simulink model "Last_Model_Interior_team"  (R2017b)
settings: Solver=VariableStepAuto  SolverName=FixedStepDiscrete  StartTime=0.0  StopTime=10  FixedStep=1e-6
PreLoadFcn:
  | %% Motor Parameters
  | Rs=6.9*10^-3;
  | Ld=220*10^-6;
  | Lq=265.4*10^-6;
  | Pm=87.78*10^-3;
  | P=4;
  | b=0.0019;
  | J=0.13;
  | f=50;
  | P_Rated=100000;
  | N_Rated=6320;
  | N_max=30000;
  | Tfl=P_Rated/(N_Rated*(2*pi/60));
  | Tl=0;
  | 
  | %% hardware impl
  | Vdc=340;
  | clocking=100;
  | fs=10000;
  | Ts=1/fs;
  | Irated=500;
  | Imax=500;
  | Id_MAX=-(Pm/Ld);
  | I_Limit=Irated;
  | I_fw=I_Limit;
  | Vmax=Vdc/sqrt(3);
  | update=2;
  | 
  | 
  | %% Inverter
  | Vdc=340;
  | deadtime=1e-6;
  | 
  | 
  | 
  | %% Tuning OF Id_Pole_Placment
  | zeta_Id=0.707;
  | Gamma_Id=0.9;
  | Wn_Id=(1/(1-Gamma_Id))*(Rs/Ld);
  | Kc_Id=(2*zeta_Id*Ld*Wn_Id)-Rs;
  | TAW_Id=((2*zeta_Id*Wn_Id*Ld)-Rs)/(Ld*Wn_Id*Wn_Id);
  | 
  | %% Tuning OF Iq_Pole_Placment
  | zeta_Iq=0.707;
  | Gamma_Iq=0.9;
  | Wn_Iq=(1/(1-Gamma_Iq))*(Rs/Lq);
  | Kc_Iq=(2*zeta_Iq*Lq*Wn_Iq)-Rs;
  | TAW_Iq=((2*zeta_Iq*Wn_Iq*Lq)-Rs)/(Lq*Wn_Iq*Wn_Iq);
  | 
  | 
  | 
  | %% Tuning of PI Using Symmetric Optimum For q phase
  | Tc=(1/fs)/update;
  | A=8;
  | Kp_SO_q=Lq/(A*(Tc)*1.5);
  | Ki_SO_q=1/((A^2)*1.5*Tc);
  | %% Tuning of PI Using Symmetric Optimum For d phase
  | Kp_SO_d=Ld/(A*(Tc)*1.5);
  | Ki_SO_d=1/((A^2)*1.5*Tc);
  | 
  | ... (+20 lines)
InitFcn:
  | %% Motor Parameters
  | Rs=6.9*10^-3;
  | Ld=220*10^-6;
  | Lq=265.4*10^-6;
  | Pm=87.78*10^-3;
  | P=4;
  | b=0.0019;
  | J=0.13;
  | f=50;
  | P_Rated=100000;
  | N_Rated=6320;
  | N_max=30000;
  | Tfl=P_Rated/(N_Rated*(2*pi/60));
  | Tl=0;
  | 
  | %% hardware impl
  | Vdc=340;
  | clocking=100;
  | fs=10000;
  | Ts=1/fs;
  | Irated=500;
  | Imax=500;
  | Id_MAX=-(Pm/Ld);
  | I_Limit=Irated;
  | I_fw=I_Limit;
  | Vmax=Vdc/sqrt(3);
  | update=2;
  | 
  | %% Inverter
  | Vdc=340;
  | deadtime=1e-6;
  | 
  | 
  | 
  | %% Tuning OF Id_Pole_Placment
  | zeta_Id=0.707;
  | Gamma_Id=0.9;
  | Wn_Id=(1/(1-Gamma_Id))*(Rs/Ld);
  | Kc_Id=(2*zeta_Id*Ld*Wn_Id)-Rs;
  | TAW_Id=((2*zeta_Id*Wn_Id*Ld)-Rs)/(Ld*Wn_Id*Wn_Id);
  | 
  | %% Tuning OF Iq_Pole_Placment
  | zeta_Iq=0.707;
  | Gamma_Iq=0.9;
  | Wn_Iq=(1/(1-Gamma_Iq))*(Rs/Lq);
  | Kc_Iq=(2*zeta_Iq*Lq*Wn_Iq)-Rs;
  | TAW_Iq=((2*zeta_Iq*Wn_Iq*Lq)-Rs)/(Lq*Wn_Iq*Wn_Iq);
  | 
  | 
  | 
  | %% Tuning of PI Using Symmetric Optimum For q phase
  | Tc=(1/fs)/update;
  | A=8;
  | Kp_SO_q=Lq/(A*(Tc)*1.5);
  | Ki_SO_q=1/((A^2)*1.5*Tc);
  | %% Tuning of PI Using Symmetric Optimum For d phase
  | Kp_SO_d=Ld/(A*(Tc)*1.5);
  | Ki_SO_d=1/((A^2)*1.5*Tc);
  | 
  | 
  | ... (+19 lines)
undefined symbols (not defined in the file): DiscIntNeverNeededParam, magnitude
libraries: simulink x81, powerlib x14
(part 3 of 4)

== system Last_Model_Interior_team/Switching/30_deg_Dpwm/Sector2 ==
  Vabc : Inport
  Enable : EnablePort
  Compare To Zero : simulink/Logic and Bit Operations/Compare To Zero  relop=<  OutDataTypeStr=boolean
  Compare To Zero1 : simulink/Logic and Bit Operations/Compare To Zero  relop=>=  OutDataTypeStr=boolean
  Demux : Demux  Outputs=3
  Enabled Subsystem : Subsystem  TreatAsAtomicUnit=on
  Enabled Subsystem1 : Subsystem  TreatAsAtomicUnit=on
  Merge : Merge
  Terminator : Terminator
  Terminator1 : Terminator
  Out1 : Outport
  wires:
  Demux/1 -> Terminator/1
  Compare To Zero/1 -> Enabled Subsystem/Enable
  Compare To Zero1/1 -> Enabled Subsystem1/Enable
  Enabled Subsystem/1(Out1) -> Merge/1
  Enabled Subsystem1/1(Out1) -> Merge/2
  Merge/1 -> Out1/1
  Vabc/1 -> Enabled Subsystem1/1(Vabc), Enabled Subsystem/1(Vabc), Demux/1
  Demux/2 -> Compare To Zero1/1, Compare To Zero/1
  Demux/3 -> Terminator1/1

== system Last_Model_Interior_team/Switching/30_deg_Dpwm/Sector3 ==
  Vabc : Inport
  Enable : EnablePort
  Compare To Zero : simulink/Logic and Bit Operations/Compare To Zero  relop=<  OutDataTypeStr=boolean
  Compare To Zero1 : simulink/Logic and Bit Operations/Compare To Zero  relop=>=  OutDataTypeStr=boolean
  Demux : Demux  Outputs=3
  Enabled Subsystem : Subsystem  TreatAsAtomicUnit=on
  Enabled Subsystem1 : Subsystem  TreatAsAtomicUnit=on
  Merge : Merge
  Terminator : Terminator
  Terminator1 : Terminator
  Out1 : Outport
  wires:
  Demux/2 -> Terminator1/1
  Demux/3 -> Compare To Zero/1, Compare To Zero1/1
  Vabc/1 -> Demux/1, Enabled Subsystem/1(Vabc), Enabled Subsystem1/1(Vabc)
  Merge/1 -> Out1/1
  Enabled Subsystem1/1(Out1) -> Merge/2
  Enabled Subsystem/1(Out1) -> Merge/1
  Compare To Zero1/1 -> Enabled Subsystem1/Enable
  Compare To Zero/1 -> Enabled Subsystem/Enable
  Demux/1 -> Terminator/1

== system Last_Model_Interior_team/Switching/30_deg_Dpwm/Sector4 ==
  Vabc : Inport
  Enable : EnablePort
  Compare To Zero : simulink/Logic and Bit Operations/Compare To Zero  relop=<  OutDataTypeStr=boolean
  Compare To Zero1 : simulink/Logic and Bit Operations/Compare To Zero  relop=>=  OutDataTypeStr=boolean
  Demux : Demux  Outputs=3
  Enabled Subsystem : Subsystem  TreatAsAtomicUnit=on
  Enabled Subsystem1 : Subsystem  TreatAsAtomicUnit=on
  Merge : Merge
  Terminator : Terminator
  Terminator1 : Terminator
  Out1 : Outport
  wires:
  Demux/3 -> Terminator/1
  Demux/1 -> Compare To Zero/1, Compare To Zero1/1
  Compare To Zero/1 -> Enabled Subsystem/Enable
  Compare To Zero1/1 -> Enabled Subsystem1/Enable
  Enabled Subsystem/1(Out1) -> Merge/1
  Enabled Subsystem1/1(Out1) -> Merge/2
  Merge/1 -> Out1/1
  Vabc/1 -> Enabled Subsystem/1(Vabc), Enabled Subsystem1/1(Vabc), Demux/1
  Demux/2 -> Terminator1/1

== system Last_Model_Interior_team/Switching/30_deg_Dpwm/Sector5 ==
  Vabc : Inport
  Enable : EnablePort
  Compare To Zero : simulink/Logic and Bit Operations/Compare To Zero  relop=<  OutDataTypeStr=boolean
  Compare To Zero1 : simulink/Logic and Bit Operations/Compare To Zero  relop=>=  OutDataTypeStr=boolean
  Demux : Demux  Outputs=3
  Enabled Subsystem : Subsystem  TreatAsAtomicUnit=on
  Enabled Subsystem1 : Subsystem  TreatAsAtomicUnit=on
  Merge : Merge
  Terminator : Terminator
  Terminator1 : Terminator
  Out1 : Outport
  wires:
  Demux/1 -> Terminator1/1
  Demux/2 -> Compare To Zero1/1, Compare To Zero/1
  Vabc/1 -> Demux/1, Enabled Subsystem1/1(Vabc), Enabled Subsystem/1(Vabc)
  Merge/1 -> Out1/1
  Enabled Subsystem1/1(Out1) -> Merge/2
  Enabled Subsystem/1(Out1) -> Merge/1
  Compare To Zero1/1 -> Enabled Subsystem1/Enable
  Compare To Zero/1 -> Enabled Subsystem/Enable
  Demux/3 -> Terminator/1

== system Last_Model_Interior_team/Switching/30_deg_Dpwm/Sector6 ==
  Vabc : Inport
  Enable : EnablePort
  Compare To Zero : simulink/Logic and Bit Operations/Compare To Zero  relop=<  OutDataTypeStr=boolean
  Compare To Zero1 : simulink/Logic and Bit Operations/Compare To Zero  relop=>=  OutDataTypeStr=boolean
  Demux : Demux  Outputs=3
  Enabled Subsystem : Subsystem  TreatAsAtomicUnit=on
  Enabled Subsystem1 : Subsystem  TreatAsAtomicUnit=on
  Merge : Merge
  Terminator : Terminator
  Terminator1 : Terminator
  Out1 : Outport
  wires:
  Demux/3 -> Compare To Zero/1, Compare To Zero1/1
  Compare To Zero/1 -> Enabled Subsystem/Enable
  Compare To Zero1/1 -> Enabled Subsystem1/Enable
  Enabled Subsystem/1(Out1) -> Merge/1
  Enabled Subsystem1/1(Out1) -> Merge/2
  Merge/1 -> Out1/1
  Vabc/1 -> Enabled Subsystem/1(Vabc), Enabled Subsystem1/1(Vabc), Demux/1
  Demux/1 -> Terminator1/1
  Demux/2 -> Terminator/1

== system Last_Model_Interior_team/Switching/60deg_+30_shifted/Sector1 ==
  Vabc : Inport
  Enable : EnablePort
  Compare To Zero : simulink/Logic and Bit Operations/Compare To Zero  relop=<  OutDataTypeStr=boolean
  Compare To Zero1 : simulink/Logic and Bit Operations/Compare To Zero  relop=>=  OutDataTypeStr=boolean
  Demux : Demux  Outputs=3
  Enabled Subsystem : Subsystem  TreatAsAtomicUnit=on
  Enabled Subsystem1 : Subsystem  TreatAsAtomicUnit=on
  Merge : Merge
  Terminator : Terminator
  Terminator1 : Terminator
  Out1 : Outport
  wires:
  Compare To Zero/1 -> Enabled Subsystem/Enable
  Compare To Zero1/1 -> Enabled Subsystem1/Enable
  Enabled Subsystem/1(Out1) -> Merge/1
  Enabled Subsystem1/1(Out1) -> Merge/2
  Merge/1 -> Out1/1
  Vabc/1 -> Enabled Subsystem/1(Vabc), Enabled Subsystem1/1(Vabc), Demux/1
  Demux/1 -> Compare To Zero1/1, Compare To Zero/1
  Demux/2 -> Terminator/1
  Demux/3 -> Terminator1/1

== system Last_Model_Interior_team/Switching/60deg_+30_shifted/Sector2 ==
  Vabc : Inport
  Enable : EnablePort
  Compare To Zero : simulink/Logic and Bit Operations/Compare To Zero  relop=<  OutDataTypeStr=boolean
  Compare To Zero1 : simulink/Logic and Bit Operations/Compare To Zero  relop=>=  OutDataTypeStr=boolean
  Demux : Demux  Outputs=3
  Enabled Subsystem : Subsystem  TreatAsAtomicUnit=on
  Enabled Subsystem1 : Subsystem  TreatAsAtomicUnit=on
  Merge : Merge
  Terminator : Terminator
  Terminator1 : Terminator
  Out1 : Outport
  wires:
  Demux/3 -> Terminator1/1
  Demux/2 -> Compare To Zero1/1, Compare To Zero/1
  Vabc/1 -> Demux/1, Enabled Subsystem/1(Vabc), Enabled Subsystem1/1(Vabc)
  Merge/1 -> Out1/1
  Enabled Subsystem1/1(Out1) -> Merge/2
  Enabled Subsystem/1(Out1) -> Merge/1
  Compare To Zero1/1 -> Enabled Subsystem1/Enable
  Compare To Zero/1 -> Enabled Subsystem/Enable
  Demux/1 -> Terminator/1

== system Last_Model_Interior_team/Switching/60deg_+30_shifted/Sector3 ==
  Vabc : Inport
  Enable : EnablePort
  Compare To Zero : simulink/Logic and Bit Operations/Compare To Zero  relop=<  OutDataTypeStr=boolean
  Compare To Zero1 : simulink/Logic and Bit Operations/Compare To Zero  relop=>=  OutDataTypeStr=boolean
  Demux : Demux  Outputs=3
  Enabled Subsystem : Subsystem  TreatAsAtomicUnit=on
  Enabled Subsystem1 : Subsystem  TreatAsAtomicUnit=on
  Merge : Merge
  Terminator : Terminator
  Terminator1 : Terminator
  Out1 : Outport
  wires:
  Demux/1 -> Terminator/1
  Compare To Zero/1 -> Enabled Subsystem/Enable
  Compare To Zero1/1 -> Enabled Subsystem1/Enable
  Enabled Subsystem/1(Out1) -> Merge/1
  Enabled Subsystem1/1(Out1) -> Merge/2
  Merge/1 -> Out1/1
  Vabc/1 -> Enabled Subsystem1/1(Vabc), Enabled Subsystem/1(Vabc), Demux/1
  Demux/3 -> Compare To Zero1/1, Compare To Zero/1
  Demux/2 -> Terminator1/1

== system Last_Model_Interior_team/Switching/60deg_+30_shifted/Sector4 ==
  Vabc : Inport
  Enable : EnablePort
  Compare To Zero : simulink/Logic and Bit Operations/Compare To Zero  relop=<  OutDataTypeStr=boolean
  Compare To Zero1 : simulink/Logic and Bit Operations/Compare To Zero  relop=>=  OutDataTypeStr=boolean
  Demux : Demux  Outputs=3
  Enabled Subsystem : Subsystem  TreatAsAtomicUnit=on
  Enabled Subsystem1 : Subsystem  TreatAsAtomicUnit=on
  Merge : Merge
  Terminator : Terminator
  Terminator1 : Terminator
  Out1 : Outport
  wires:
  Demux/2 -> Terminator1/1
  Vabc/1 -> Demux/1, Enabled Subsystem1/1(Vabc), Enabled Subsystem/1(Vabc)
  Merge/1 -> Out1/1
  Enabled Subsystem1/1(Out1) -> Merge/2
  Enabled Subsystem/1(Out1) -> Merge/1
  Compare To Zero1/1 -> Enabled Subsystem1/Enable
  Compare To Zero/1 -> Enabled Subsystem/Enable
  Demux/1 -> Compare To Zero1/1, Compare To Zero/1
  Demux/3 -> Terminator/1

== system Last_Model_Interior_team/Switching/60deg_+30_shifted/Sector5 ==
  Vabc : Inport
  Enable : EnablePort
  Compare To Zero : simulink/Logic and Bit Operations/Compare To Zero  relop=<  OutDataTypeStr=boolean
  Compare To Zero1 : simulink/Logic and Bit Operations/Compare To Zero  relop=>=  OutDataTypeStr=boolean
  Demux : Demux  Outputs=3
  Enabled Subsystem : Subsystem  TreatAsAtomicUnit=on
  Enabled Subsystem1 : Subsystem  TreatAsAtomicUnit=on
  Merge : Merge
  Terminator : Terminator
  Terminator1 : Terminator
  Out1 : Outport
  wires:
  Demux/3 -> Terminator/1
  Compare To Zero/1 -> Enabled Subsystem/Enable
  Compare To Zero1/1 -> Enabled Subsystem1/Enable
  Enabled Subsystem/1(Out1) -> Merge/1
  Enabled Subsystem1/1(Out1) -> Merge/2
  Merge/1 -> Out1/1
  Vabc/1 -> Enabled Subsystem/1(Vabc), Enabled Subsystem1/1(Vabc), Demux/1
  Demux/2 -> Compare To Zero/1, Compare To Zero1/1
  Demux/1 -> Terminator1/1

== system Last_Model_Interior_team/Switching/60deg_+30_shifted/Sector6 ==
  Vabc : Inport
  Enable : EnablePort
  Compare To Zero : simulink/Logic and Bit Operations/Compare To Zero  relop=<  OutDataTypeStr=boolean
  Compare To Zero1 : simulink/Logic and Bit Operations/Compare To Zero  relop=>=  OutDataTypeStr=boolean
  Demux : Demux  Outputs=3
  Enabled Subsystem : Subsystem  TreatAsAtomicUnit=on
  Enabled Subsystem1 : Subsystem  TreatAsAtomicUnit=on
  Merge : Merge
  Terminator : Terminator
  Terminator1 : Terminator
  Out1 : Outport
  wires:
  Demux/1 -> Terminator1/1
  Vabc/1 -> Demux/1, Enabled Subsystem1/1(Vabc), Enabled Subsystem/1(Vabc)
  Merge/1 -> Out1/1
  Enabled Subsystem1/1(Out1) -> Merge/2
  Enabled Subsystem/1(Out1) -> Merge/1
  Compare To Zero1/1 -> Enabled Subsystem1/Enable
  Compare To Zero/1 -> Enabled Subsystem/Enable
  Demux/3 -> Compare To Zero1/1, Compare To Zero/1
  Demux/2 -> Terminator/1

== system Last_Model_Interior_team/Switching/60deg_-30_shifted/Sector1 ==
  Vabc : Inport
  Enable : EnablePort
  Compare To Zero : simulink/Logic and Bit Operations/Compare To Zero  relop=<  OutDataTypeStr=boolean
  Compare To Zero1 : simulink/Logic and Bit Operations/Compare To Zero  relop=>=  OutDataTypeStr=boolean
  Demux : Demux  Outputs=3
  Enabled Subsystem : Subsystem  TreatAsAtomicUnit=on
  Enabled Subsystem1 : Subsystem  TreatAsAtomicUnit=on
  Merge : Merge
  Terminator : Terminator
  Terminator1 : Terminator
  Out1 : Outport
  wires:
  Demux/3 -> Terminator1/1
  Demux/2 -> Terminator/1
  Demux/1 -> Compare To Zero/1, Compare To Zero1/1
  Vabc/1 -> Demux/1, Enabled Subsystem1/1(Vabc), Enabled Subsystem/1(Vabc)
  Merge/1 -> Out1/1
  Enabled Subsystem1/1(Out1) -> Merge/2
  Enabled Subsystem/1(Out1) -> Merge/1
  Compare To Zero1/1 -> Enabled Subsystem1/Enable
  Compare To Zero/1 -> Enabled Subsystem/Enable

== system Last_Model_Interior_team/Switching/60deg_-30_shifted/Sector2 ==
  Vabc : Inport
  Enable : EnablePort
  Compare To Zero : simulink/Logic and Bit Operations/Compare To Zero  relop=<  OutDataTypeStr=boolean
  Compare To Zero1 : simulink/Logic and Bit Operations/Compare To Zero  relop=>=  OutDataTypeStr=boolean
  Demux : Demux  Outputs=3
  Enabled Subsystem : Subsystem  TreatAsAtomicUnit=on
  Enabled Subsystem1 : Subsystem  TreatAsAtomicUnit=on
  Merge : Merge
  Terminator : Terminator
  Terminator1 : Terminator
  Out1 : Outport
  wires:
  Demux/1 -> Terminator/1
  Compare To Zero/1 -> Enabled Subsystem/Enable
  Compare To Zero1/1 -> Enabled Subsystem1/Enable
  Enabled Subsystem/1(Out1) -> Merge/1
  Enabled Subsystem1/1(Out1) -> Merge/2
  Merge/1 -> Out1/1
  Vabc/1 -> Enabled Subsystem1/1(Vabc), Enabled Subsystem/1(Vabc), Demux/1
  Demux/2 -> Compare To Zero/1, Compare To Zero1/1
  Demux/3 -> Terminator1/1

== system Last_Model_Interior_team/Switching/60deg_-30_shifted/Sector3 ==
  Vabc : Inport
  Enable : EnablePort
  Compare To Zero : simulink/Logic and Bit Operations/Compare To Zero  relop=<  OutDataTypeStr=boolean
  Compare To Zero1 : simulink/Logic and Bit Operations/Compare To Zero  relop=>=  OutDataTypeStr=boolean
  Demux : Demux  Outputs=3
  Enabled Subsystem : Subsystem  TreatAsAtomicUnit=on
  Enabled Subsystem1 : Subsystem  TreatAsAtomicUnit=on
  Merge : Merge
  Terminator : Terminator
  Terminator1 : Terminator
  Out1 : Outport
  wires:
  Demux/2 -> Terminator1/1
  Demux/3 -> Compare To Zero/1, Compare To Zero1/1
  Vabc/1 -> Demux/1, Enabled Subsystem/1(Vabc), Enabled Subsystem1/1(Vabc)
  Merge/1 -> Out1/1
  Enabled Subsystem1/1(Out1) -> Merge/2
  Enabled Subsystem/1(Out1) -> Merge/1
  Compare To Zero1/1 -> Enabled Subsystem1/Enable
  Compare To Zero/1 -> Enabled Subsystem/Enable
  Demux/1 -> Terminator/1

== system Last_Model_Interior_team/Switching/60deg_-30_shifted/Sector4 ==
  Vabc : Inport
  Enable : EnablePort
  Compare To Zero : simulink/Logic and Bit Operations/Compare To Zero  relop=<  OutDataTypeStr=boolean
  Compare To Zero1 : simulink/Logic and Bit Operations/Compare To Zero  relop=>=  OutDataTypeStr=boolean
  Demux : Demux  Outputs=3
  Enabled Subsystem : Subsystem  TreatAsAtomicUnit=on
  Enabled Subsystem1 : Subsystem  TreatAsAtomicUnit=on
  Merge : Merge
  Terminator : Terminator
  Terminator1 : Terminator
  Out1 : Outport
  wires:
  Demux/3 -> Terminator/1
  Demux/1 -> Compare To Zero/1, Compare To Zero1/1
  Compare To Zero/1 -> Enabled Subsystem/Enable
  Compare To Zero1/1 -> Enabled Subsystem1/Enable
  Enabled Subsystem/1(Out1) -> Merge/1
  Enabled Subsystem1/1(Out1) -> Merge/2
  Merge/1 -> Out1/1
  Vabc/1 -> Enabled Subsystem/1(Vabc), Enabled Subsystem1/1(Vabc), Demux/1
  Demux/2 -> Terminator1/1

== system Last_Model_Interior_team/Switching/60deg_-30_shifted/Sector5 ==
  Vabc : Inport
  Enable : EnablePort
  Compare To Zero : simulink/Logic and Bit Operations/Compare To Zero  relop=<  OutDataTypeStr=boolean
  Compare To Zero1 : simulink/Logic and Bit Operations/Compare To Zero  relop=>=  OutDataTypeStr=boolean
  Demux : Demux  Outputs=3
  Enabled Subsystem : Subsystem  TreatAsAtomicUnit=on
  Enabled Subsystem1 : Subsystem  TreatAsAtomicUnit=on
  Merge : Merge
  Terminator : Terminator
  Terminator1 : Terminator
  Out1 : Outport
  wires:
  Demux/1 -> Terminator1/1
  Demux/2 -> Compare To Zero1/1, Compare To Zero/1
  Vabc/1 -> Demux/1, Enabled Subsystem1/1(Vabc), Enabled Subsystem/1(Vabc)
  Merge/1 -> Out1/1
  Enabled Subsystem1/1(Out1) -> Merge/2
  Enabled Subsystem/1(Out1) -> Merge/1
  Compare To Zero1/1 -> Enabled Subsystem1/Enable
  Compare To Zero/1 -> Enabled Subsystem/Enable
  Demux/3 -> Terminator/1

== system Last_Model_Interior_team/Switching/60deg_-30_shifted/Sector6 ==
  Vabc : Inport
  Enable : EnablePort
  Compare To Zero : simulink/Logic and Bit Operations/Compare To Zero  relop=<  OutDataTypeStr=boolean
  Compare To Zero1 : simulink/Logic and Bit Operations/Compare To Zero  relop=>=  OutDataTypeStr=boolean
  Demux : Demux  Outputs=3
  Enabled Subsystem : Subsystem  TreatAsAtomicUnit=on
  Enabled Subsystem1 : Subsystem  TreatAsAtomicUnit=on
  Merge : Merge
  Terminator : Terminator
  Terminator1 : Terminator
  Out1 : Outport
  wires:
  Demux/2 -> Terminator/1
  Demux/3 -> Compare To Zero/1, Compare To Zero1/1
  Compare To Zero/1 -> Enabled Subsystem/Enable
  Compare To Zero1/1 -> Enabled Subsystem1/Enable
  Enabled Subsystem/1(Out1) -> Merge/1
  Enabled Subsystem1/1(Out1) -> Merge/2
  Merge/1 -> Out1/1
  Vabc/1 -> Enabled Subsystem/1(Vabc), Enabled Subsystem1/1(Vabc), Demux/1
  Demux/1 -> Terminator1/1

== system Last_Model_Interior_team/Switching/60deg_DPWM/Sector1 ==
  Vabc : Inport
  Enable : EnablePort
  Compare To Zero : simulink/Logic and Bit Operations/Compare To Zero  relop=<  OutDataTypeStr=boolean
  Compare To Zero1 : simulink/Logic and Bit Operations/Compare To Zero  relop=>=  OutDataTypeStr=boolean
  Demux : Demux  Outputs=3
  Enabled Subsystem : Subsystem  TreatAsAtomicUnit=on
  Enabled Subsystem1 : Subsystem  TreatAsAtomicUnit=on
  Merge : Merge
  Terminator : Terminator
  Terminator1 : Terminator
  Out1 : Outport
  wires:
  Enabled Subsystem/1(Out1) -> Merge/1
  Enabled Subsystem1/1(Out1) -> Merge/2
  Merge/1 -> Out1/1
  Vabc/1 -> Enabled Subsystem/1(Vabc), Enabled Subsystem1/1(Vabc), Demux/1
  Demux/1 -> Compare To Zero1/1, Compare To Zero/1
  Demux/2 -> Terminator/1
  Demux/3 -> Terminator1/1
  Compare To Zero1/1 -> Enabled Subsystem1/Enable
  Compare To Zero/1 -> Enabled Subsystem/Enable

== system Last_Model_Interior_team/Switching/60deg_DPWM/Sector2 ==
  Vabc : Inport
  Enable : EnablePort
  Compare To Zero : simulink/Logic and Bit Operations/Compare To Zero  relop=<  OutDataTypeStr=boolean
  Compare To Zero1 : simulink/Logic and Bit Operations/Compare To Zero  relop=>=  OutDataTypeStr=boolean
  Demux : Demux  Outputs=3
  Enabled Subsystem : Subsystem  TreatAsAtomicUnit=on
  Enabled Subsystem1 : Subsystem  TreatAsAtomicUnit=on
  Merge : Merge
  Terminator : Terminator
  Terminator1 : Terminator
  Out1 : Outport
  wires:
  Demux/3 -> Terminator1/1
  Demux/2 -> Compare To Zero1/1, Compare To Zero/1
  Vabc/1 -> Demux/1, Enabled Subsystem1/1(Vabc), Enabled Subsystem/1(Vabc)
  Merge/1 -> Out1/1
  Enabled Subsystem1/1(Out1) -> Merge/2
  Enabled Subsystem/1(Out1) -> Merge/1
  Compare To Zero1/1 -> Enabled Subsystem1/Enable
  Compare To Zero/1 -> Enabled Subsystem/Enable
  Demux/1 -> Terminator/1

== system Last_Model_Interior_team/Switching/60deg_DPWM/Sector3 ==
  Vabc : Inport
  Enable : EnablePort
  Compare To Zero : simulink/Logic and Bit Operations/Compare To Zero  relop=<  OutDataTypeStr=boolean
  Compare To Zero1 : simulink/Logic and Bit Operations/Compare To Zero  relop=>=  OutDataTypeStr=boolean
  Demux : Demux  Outputs=3
  Enabled Subsystem : Subsystem  TreatAsAtomicUnit=on
  Enabled Subsystem1 : Subsystem  TreatAsAtomicUnit=on
  Merge : Merge
  Terminator : Terminator
  Terminator1 : Terminator
  Out1 : Outport
  wires:
  Demux/1 -> Terminator/1
  Compare To Zero/1 -> Enabled Subsystem/Enable
  Compare To Zero1/1 -> Enabled Subsystem1/Enable
  Enabled Subsystem/1(Out1) -> Merge/1
  Enabled Subsystem1/1(Out1) -> Merge/2
  Merge/1 -> Out1/1
  Vabc/1 -> Enabled Subsystem/1(Vabc), Enabled Subsystem1/1(Vabc), Demux/1
  Demux/3 -> Compare To Zero1/1, Compare To Zero/1
  Demux/2 -> Terminator1/1

== system Last_Model_Interior_team/Switching/60deg_DPWM/Sector4 ==
  Vabc : Inport
  Enable : EnablePort
  Compare To Zero : simulink/Logic and Bit Operations/Compare To Zero  relop=<  OutDataTypeStr=boolean
  Compare To Zero1 : simulink/Logic and Bit Operations/Compare To Zero  relop=>=  OutDataTypeStr=boolean
  Demux : Demux  Outputs=3
  Enabled Subsystem : Subsystem  TreatAsAtomicUnit=on
  Enabled Subsystem1 : Subsystem  TreatAsAtomicUnit=on
  Merge : Merge
  Terminator : Terminator
  Terminator1 : Terminator
  Out1 : Outport
  wires:
  Demux/2 -> Terminator1/1
  Vabc/1 -> Demux/1, Enabled Subsystem1/1(Vabc), Enabled Subsystem/1(Vabc)
  Merge/1 -> Out1/1
  Enabled Subsystem1/1(Out1) -> Merge/2
  Enabled Subsystem/1(Out1) -> Merge/1
  Compare To Zero1/1 -> Enabled Subsystem1/Enable
  Compare To Zero/1 -> Enabled Subsystem/Enable
  Demux/1 -> Compare To Zero1/1, Compare To Zero/1
  Demux/3 -> Terminator/1

== system Last_Model_Interior_team/Switching/60deg_DPWM/Sector5 ==
  Vabc : Inport
  Enable : EnablePort
  Compare To Zero : simulink/Logic and Bit Operations/Compare To Zero  relop=<  OutDataTypeStr=boolean
  Compare To Zero1 : simulink/Logic and Bit Operations/Compare To Zero  relop=>=  OutDataTypeStr=boolean
  Demux : Demux  Outputs=3
  Enabled Subsystem : Subsystem  TreatAsAtomicUnit=on
  Enabled Subsystem1 : Subsystem  TreatAsAtomicUnit=on
  Merge : Merge
  Terminator : Terminator
  Terminator1 : Terminator
  Out1 : Outport
  wires:
  Demux/3 -> Terminator/1
  Compare To Zero/1 -> Enabled Subsystem/Enable
  Compare To Zero1/1 -> Enabled Subsystem1/Enable
  Enabled Subsystem/1(Out1) -> Merge/1
  Enabled Subsystem1/1(Out1) -> Merge/2
  Merge/1 -> Out1/1
  Vabc/1 -> Enabled Subsystem/1(Vabc), Enabled Subsystem1/1(Vabc), Demux/1
  Demux/2 -> Compare To Zero/1, Compare To Zero1/1
  Demux/1 -> Terminator1/1

== system Last_Model_Interior_team/Switching/60deg_DPWM/Sector6 ==
  Vabc : Inport
  Enable : EnablePort
  Compare To Zero : simulink/Logic and Bit Operations/Compare To Zero  relop=<  OutDataTypeStr=boolean
  Compare To Zero1 : simulink/Logic and Bit Operations/Compare To Zero  relop=>=  OutDataTypeStr=boolean
  Demux : Demux  Outputs=3
  Enabled Subsystem : Subsystem  TreatAsAtomicUnit=on
  Enabled Subsystem1 : Subsystem  TreatAsAtomicUnit=on
  Merge : Merge
  Terminator : Terminator
  Terminator1 : Terminator
  Out1 : Outport
  wires:
  Demux/1 -> Terminator1/1
  Vabc/1 -> Demux/1, Enabled Subsystem1/1(Vabc), Enabled Subsystem/1(Vabc)
  Merge/1 -> Out1/1
  Enabled Subsystem1/1(Out1) -> Merge/2
  Enabled Subsystem/1(Out1) -> Merge/1
  Compare To Zero1/1 -> Enabled Subsystem1/Enable
  Compare To Zero/1 -> Enabled Subsystem/Enable
  Demux/3 -> Compare To Zero1/1, Compare To Zero/1
  Demux/2 -> Terminator/1

== system Last_Model_Interior_team/Flux_Weakening/Region_2/Subsystem/Zero detection ==
  In1 : Inport
  Constant : Constant  Value=eps
  Switch : Switch  Criteria=u2 > Threshold  Threshold=eps
  Out1 : Outport
  wires:
  Switch/1 -> Out1/1
  Constant/1 -> Switch/3
  In1/1 -> Switch/2, Switch/1

== system Last_Model_Interior_team/Switching/+120_deg_Dpwm/Sector1/Enabled Subsystem ==
  Vabc : Inport
  Enable : EnablePort
  Add : Sum  Inputs=-+
  Constant : Constant
  Demux : Demux  Outputs=3
  Terminator : Terminator
  Terminator1 : Terminator
  Out1 : Outport
  wires:
  Add/1 -> Out1/1
  Demux/2 -> Add/1
  Demux/3 -> Terminator1/1
  Vabc/1 -> Demux/1
  Constant/1 -> Add/2
  Demux/1 -> Terminator/1

== system Last_Model_Interior_team/Switching/+120_deg_Dpwm/Sector1/Enabled Subsystem1 ==
  Vabc : Inport
  Enable : EnablePort
  Add : Sum  Inputs=-+
  Constant : Constant
  Demux : Demux  Outputs=3
  Terminator : Terminator
  Terminator1 : Terminator
  Out1 : Outport
  wires:
  Demux/1 -> Terminator/1
  Constant/1 -> Add/2
  Vabc/1 -> Demux/1
  Add/1 -> Out1/1
  Demux/2 -> Add/1
  Demux/3 -> Terminator1/1

== system Last_Model_Interior_team/Switching/+120_deg_Dpwm/Sector2/Enabled Subsystem ==
  Vabc : Inport
  Enable : EnablePort
  Add : Sum  Inputs=-+
  Constant : Constant
  Demux : Demux  Outputs=3
  Terminator : Terminator
  Terminator1 : Terminator
  Out1 : Outport
  wires:
  Demux/1 -> Add/1
  Demux/2 -> Terminator/1
  Constant/1 -> Add/2
  Vabc/1 -> Demux/1
  Demux/3 -> Terminator1/1
  Add/1 -> Out1/1

== system Last_Model_Interior_team/Switching/+120_deg_Dpwm/Sector2/Enabled Subsystem1 ==
  Vabc : Inport
  Enable : EnablePort
  Add : Sum  Inputs=-+
  Constant : Constant
  Demux : Demux  Outputs=3
  Terminator : Terminator
  Terminator1 : Terminator
  Out1 : Outport
  wires:
  Add/1 -> Out1/1
  Demux/3 -> Terminator1/1
  Vabc/1 -> Demux/1
  Constant/1 -> Add/2
  Demux/2 -> Terminator/1
  Demux/1 -> Add/1

== system Last_Model_Interior_team/Switching/+120_deg_Dpwm/Sector3/Enabled Subsystem ==
  Vabc : Inport
  Enable : EnablePort
  Add : Sum  Inputs=-+
  Constant : Constant
  Demux : Demux  Outputs=3
  Terminator : Terminator
  Terminator1 : Terminator
  Out1 : Outport
  wires:
  Add/1 -> Out1/1
  Demux/3 -> Terminator1/1
  Vabc/1 -> Demux/1
  Constant/1 -> Add/2
  Demux/2 -> Terminator/1
  Demux/1 -> Add/1

== system Last_Model_Interior_team/Switching/+120_deg_Dpwm/Sector3/Enabled Subsystem1 ==
  Vabc : Inport
  Enable : EnablePort
  Add : Sum  Inputs=-+
  Constant : Constant
  Demux : Demux  Outputs=3
  Terminator : Terminator
  Terminator1 : Terminator
  Out1 : Outport
  wires:
  Demux/1 -> Add/1
  Demux/2 -> Terminator/1
  Constant/1 -> Add/2
  Vabc/1 -> Demux/1
  Demux/3 -> Terminator1/1
  Add/1 -> Out1/1

== system Last_Model_Interior_team/Switching/+120_deg_Dpwm/Sector4/Enabled Subsystem ==
  Vabc : Inport
  Enable : EnablePort
  Add : Sum  Inputs=-+
  Constant : Constant
  Demux : Demux  Outputs=3
  Terminator : Terminator
  Terminator1 : Terminator
  Out1 : Outport
  wires:
  Demux/3 -> Add/1
  Constant/1 -> Add/2
  Demux/1 -> Terminator/1
  Vabc/1 -> Demux/1
  Add/1 -> Out1/1
  Demux/2 -> Terminator1/1

== system Last_Model_Interior_team/Switching/+120_deg_Dpwm/Sector4/Enabled Subsystem1 ==
  Vabc : Inport
  Enable : EnablePort
  Add : Sum  Inputs=-+
  Constant : Constant
  Demux : Demux  Outputs=3
  Terminator : Terminator
  Terminator1 : Terminator
  Out1 : Outport
  wires:
  Vabc/1 -> Demux/1
  Demux/1 -> Terminator/1
  Constant/1 -> Add/2
  Add/1 -> Out1/1
  Demux/3 -> Add/1
  Demux/2 -> Terminator1/1

== system Last_Model_Interior_team/Switching/+120_deg_Dpwm/Sector5/Enabled Subsystem ==
  Vabc : Inport
  Enable : EnablePort
  Add : Sum  Inputs=-+
  Constant : Constant
  Demux : Demux  Outputs=3
  Terminator : Terminator
  Terminator1 : Terminator
  Out1 : Outport
  wires:
  Add/1 -> Out1/1
  Demux/3 -> Add/1
  Vabc/1 -> Demux/1
  Constant/1 -> Add/2
  Demux/2 -> Terminator/1
  Demux/1 -> Terminator1/1

== system Last_Model_Interior_team/Switching/+120_deg_Dpwm/Sector5/Enabled Subsystem1 ==
  Vabc : Inport
  Enable : EnablePort
  Add : Sum  Inputs=-+
  Constant : Constant
  Demux : Demux  Outputs=3
  Terminator : Terminator
  Terminator1 : Terminator
  Out1 : Outport
  wires:
  Add/1 -> Out1/1
  Constant/1 -> Add/2
  Demux/1 -> Terminator1/1
  Demux/2 -> Terminator/1
  Vabc/1 -> Demux/1
  Demux/3 -> Add/1

== system Last_Model_Interior_team/Switching/+120_deg_Dpwm/Sector6/Enabled Subsystem ==
  Vabc : Inport
  Enable : EnablePort
  Add : Sum  Inputs=-+
  Constant : Constant
  Demux : Demux  Outputs=3
  Terminator : Terminator
  Terminator1 : Terminator
  Out1 : Outport
  wires:
  Demux/2 -> Add/1
  Vabc/1 -> Demux/1
  Constant/1 -> Add/2
  Demux/3 -> Terminator1/1
  Add/1 -> Out1/1
  Demux/1 -> Terminator/1

== system Last_Model_Interior_team/Switching/+120_deg_Dpwm/Sector6/Enabled Subsystem1 ==
  Vabc : Inport
  Enable : EnablePort
  Add : Sum  Inputs=-+
  Constant : Constant
  Demux : Demux  Outputs=3
  Terminator : Terminator
  Terminator1 : Terminator
  Out1 : Outport
  wires:
  Vabc/1 -> Demux/1
  Constant/1 -> Add/2
  Add/1 -> Out1/1
  Demux/3 -> Terminator1/1
  Demux/2 -> Add/1
  Demux/1 -> Terminator/1

== system Last_Model_Interior_team/Switching/-120_deg_Dpwm/Sector1/Enabled Subsystem ==
  Vabc : Inport
  Enable : EnablePort
  Add : Sum  Inputs=-+
  Constant : Constant  Value=-1
  Demux : Demux  Outputs=3
  Terminator : Terminator
  Terminator1 : Terminator
  Out1 : Outport
  wires:
  Demux/1 -> Terminator/1
  Constant/1 -> Add/2
  Vabc/1 -> Demux/1
  Demux/3 -> Add/1
  Add/1 -> Out1/1
  Demux/2 -> Terminator1/1

== system Last_Model_Interior_team/Switching/-120_deg_Dpwm/Sector1/Enabled Subsystem1 ==
  Vabc : Inport
  Enable : EnablePort
  Add : Sum  Inputs=-+
  Constant : Constant  Value=-1
  Demux : Demux  Outputs=3
  Terminator : Terminator
  Terminator1 : Terminator
  Out1 : Outport
  wires:
  Add/1 -> Out1/1
  Vabc/1 -> Demux/1
  Constant/1 -> Add/2
  Demux/1 -> Terminator/1
  Demux/2 -> Terminator1/1
  Demux/3 -> Add/1

== system Last_Model_Interior_team/Switching/-120_deg_Dpwm/Sector2/Enabled Subsystem ==
  Vabc : Inport
  Enable : EnablePort
  Add : Sum  Inputs=-+
  Constant : Constant  Value=-1
  Demux : Demux  Outputs=3
  Terminator : Terminator
  Terminator1 : Terminator
  Out1 : Outport
  wires:
  Add/1 -> Out1/1
  Demux/3 -> Add/1
  Vabc/1 -> Demux/1
  Constant/1 -> Add/2
  Demux/2 -> Terminator/1
  Demux/1 -> Terminator1/1

== system Last_Model_Interior_team/Switching/-120_deg_Dpwm/Sector2/Enabled Subsystem1 ==
  Vabc : Inport
  Enable : EnablePort
  Add : Sum  Inputs=-+
  Constant : Constant  Value=-1
  Demux : Demux  Outputs=3
  Terminator : Terminator
  Terminator1 : Terminator
  Out1 : Outport
  wires:
  Demux/2 -> Terminator/1
  Constant/1 -> Add/2
  Vabc/1 -> Demux/1
  Demux/3 -> Add/1
  Add/1 -> Out1/1
  Demux/1 -> Terminator1/1

== system Last_Model_Interior_team/Switching/-120_deg_Dpwm/Sector3/Enabled Subsystem ==
  Vabc : Inport
  Enable : EnablePort
  Add : Sum  Inputs=-+
  Constant : Constant  Value=-1
  Demux : Demux  Outputs=3
  Terminator : Terminator
  Terminator1 : Terminator
  Out1 : Outport
  wires:
  Demux/2 -> Add/1
  Constant/1 -> Add/2
  Vabc/1 -> Demux/1
  Demux/3 -> Terminator1/1
  Add/1 -> Out1/1
  Demux/1 -> Terminator/1

== system Last_Model_Interior_team/Switching/-120_deg_Dpwm/Sector3/Enabled Subsystem1 ==
  Vabc : Inport
  Enable : EnablePort
  Add : Sum  Inputs=-+
  Constant : Constant  Value=-1
  Demux : Demux  Outputs=3
  Terminator : Terminator
  Terminator1 : Terminator
  Out1 : Outport
  wires:
  Add/1 -> Out1/1
  Demux/3 -> Terminator1/1
  Vabc/1 -> Demux/1
  Constant/1 -> Add/2
  Demux/2 -> Add/1
  Demux/1 -> Terminator/1

== system Last_Model_Interior_team/Switching/-120_deg_Dpwm/Sector4/Enabled Subsystem ==
  Vabc : Inport
  Enable : EnablePort
  Add : Sum  Inputs=-+
  Constant : Constant  Value=-1
  Demux : Demux  Outputs=3
  Terminator : Terminator
  Terminator1 : Terminator
  Out1 : Outport
  wires:
  Add/1 -> Out1/1
  Vabc/1 -> Demux/1
  Demux/1 -> Terminator/1
  Constant/1 -> Add/2
  Demux/3 -> Terminator1/1
  Demux/2 -> Add/1

== system Last_Model_Interior_team/Switching/-120_deg_Dpwm/Sector4/Enabled Subsystem1 ==
  Vabc : Inport
  Enable : EnablePort
  Add : Sum  Inputs=-+
  Constant : Constant  Value=-1
  Demux : Demux  Outputs=3
  Terminator : Terminator
  Terminator1 : Terminator
  Out1 : Outport
  wires:
  Demux/2 -> Add/1
  Add/1 -> Out1/1
  Constant/1 -> Add/2
  Demux/1 -> Terminator/1
  Vabc/1 -> Demux/1
  Demux/3 -> Terminator1/1

== system Last_Model_Interior_team/Switching/-120_deg_Dpwm/Sector5/Enabled Subsystem ==
  Vabc : Inport
  Enable : EnablePort
  Add : Sum  Inputs=-+
  Constant : Constant  Value=-1
  Demux : Demux  Outputs=3
  Terminator : Terminator
  Terminator1 : Terminator
  Out1 : Outport
  wires:
  Demux/2 -> Terminator/1
  Constant/1 -> Add/2
  Vabc/1 -> Demux/1
  Demux/1 -> Add/1
  Add/1 -> Out1/1
  Demux/3 -> Terminator1/1

== system Last_Model_Interior_team/Switching/-120_deg_Dpwm/Sector5/Enabled Subsystem1 ==
  Vabc : Inport
  Enable : EnablePort
  Add : Sum  Inputs=-+
  Constant : Constant  Value=-1
  Demux : Demux  Outputs=3
  Terminator : Terminator
  Terminator1 : Terminator
  Out1 : Outport
  wires:
  Demux/1 -> Add/1
  Vabc/1 -> Demux/1
  Demux/2 -> Terminator/1
  Constant/1 -> Add/2
  Add/1 -> Out1/1
  Demux/3 -> Terminator1/1

== system Last_Model_Interior_team/Switching/-120_deg_Dpwm/Sector6/Enabled Subsystem ==
  Vabc : Inport
  Enable : EnablePort
  Add : Sum  Inputs=-+
  Constant : Constant  Value=-1
  Demux : Demux  Outputs=3
  Terminator : Terminator
  Terminator1 : Terminator
  Out1 : Outport
  wires:
  Demux/3 -> Terminator1/1
  Add/1 -> Out1/1
  Demux/1 -> Add/1
  Vabc/1 -> Demux/1
  Constant/1 -> Add/2
  Demux/2 -> Terminator/1

== system Last_Model_Interior_team/Switching/-120_deg_Dpwm/Sector6/Enabled Subsystem1 ==
  Vabc : Inport
  Enable : EnablePort
  Add : Sum  Inputs=-+
  Constant : Constant  Value=-1
  Demux : Demux  Outputs=3
  Terminator : Terminator
  Terminator1 : Terminator
  Out1 : Outport
  wires:
  Demux/3 -> Terminator1/1
  Add/1 -> Out1/1
  Constant/1 -> Add/2
  Demux/2 -> Terminator/1
  Vabc/1 -> Demux/1
  Demux/1 -> Add/1

== system Last_Model_Interior_team/Switching/30_deg_Dpwm/Sector1/Enabled Subsystem ==
  Vabc : Inport
  Enable : EnablePort
  Add : Sum  Inputs=-+
  Constant : Constant  Value=-1
  Demux : Demux  Outputs=3
  Terminator : Terminator
  Terminator1 : Terminator
  Out1 : Outport
  wires:
  Demux/2 -> Terminator1/1
  Add/1 -> Out1/1
  Demux/3 -> Add/1
  Vabc/1 -> Demux/1
  Constant/1 -> Add/2
  Demux/1 -> Terminator/1

== system Last_Model_Interior_team/Switching/30_deg_Dpwm/Sector1/Enabled Subsystem1 ==
  Vabc : Inport
  Enable : EnablePort
  Add : Sum  Inputs=-+
  Constant : Constant
  Demux : Demux  Outputs=3
  Terminator : Terminator
  Terminator1 : Terminator
  Out1 : Outport
  wires:
  Demux/2 -> Add/1
  Demux/1 -> Terminator/1
  Constant/1 -> Add/2
  Vabc/1 -> Demux/1
  Add/1 -> Out1/1
  Demux/3 -> Terminator1/1

== system Last_Model_Interior_team/Switching/30_deg_Dpwm/Sector2/Enabled Subsystem ==
  Vabc : Inport
  Enable : EnablePort
  Add : Sum  Inputs=-+
  Constant : Constant  Value=-1
  Demux : Demux  Outputs=3
  Terminator : Terminator
  Terminator1 : Terminator
  Out1 : Outport
  wires:
  Demux/1 -> Terminator1/1
  Demux/2 -> Terminator/1
  Constant/1 -> Add/2
  Vabc/1 -> Demux/1
  Demux/3 -> Add/1
  Add/1 -> Out1/1

== system Last_Model_Interior_team/Switching/30_deg_Dpwm/Sector2/Enabled Subsystem1 ==
  Vabc : Inport
  Enable : EnablePort
  Add : Sum  Inputs=-+
  Constant : Constant
  Demux : Demux  Outputs=3
  Terminator : Terminator
  Terminator1 : Terminator
  Out1 : Outport
  wires:
  Demux/1 -> Add/1
  Add/1 -> Out1/1
  Vabc/1 -> Demux/1
  Constant/1 -> Add/2
  Demux/2 -> Terminator/1
  Demux/3 -> Terminator1/1

== system Last_Model_Interior_team/Switching/30_deg_Dpwm/Sector3/Enabled Subsystem ==
  Vabc : Inport
  Enable : EnablePort
  Add : Sum  Inputs=-+
  Constant : Constant  Value=-1
  Demux : Demux  Outputs=3
  Terminator : Terminator
  Terminator1 : Terminator
  Out1 : Outport
  wires:
  Demux/1 -> Terminator/1
  Add/1 -> Out1/1
  Demux/3 -> Terminator1/1
  Vabc/1 -> Demux/1
  Constant/1 -> Add/2
  Demux/2 -> Add/1

== system Last_Model_Interior_team/Switching/30_deg_Dpwm/Sector3/Enabled Subsystem1 ==
  Vabc : Inport
  Enable : EnablePort
  Add : Sum  Inputs=-+
  Constant : Constant
  Demux : Demux  Outputs=3
  Terminator : Terminator
  Terminator1 : Terminator
  Out1 : Outport
  wires:
  Demux/1 -> Add/1
  Constant/1 -> Add/2
  Vabc/1 -> Demux/1
  Demux/3 -> Terminator1/1
  Add/1 -> Out1/1
  Demux/2 -> Terminator/1

== system Last_Model_Interior_team/Switching/30_deg_Dpwm/Sector4/Enabled Subsystem ==
  Vabc : Inport
  Enable : EnablePort
  Add : Sum  Inputs=-+
  Constant : Constant  Value=-1
  Demux : Demux  Outputs=3
  Terminator : Terminator
  Terminator1 : Terminator
  Out1 : Outport
  wires:
  Demux/2 -> Add/1
  Demux/3 -> Terminator1/1
  Constant/1 -> Add/2
  Demux/1 -> Terminator/1
  Vabc/1 -> Demux/1
  Add/1 -> Out1/1

== system Last_Model_Interior_team/Switching/30_deg_Dpwm/Sector4/Enabled Subsystem1 ==
  Vabc : Inport
  Enable : EnablePort
  Add : Sum  Inputs=-+
  Constant : Constant
  Demux : Demux  Outputs=3
  Terminator : Terminator
  Terminator1 : Terminator
  Out1 : Outport
  wires:
  Demux/3 -> Add/1
  Vabc/1 -> Demux/1
  Demux/1 -> Terminator/1
  Constant/1 -> Add/2
  Add/1 -> Out1/1
  Demux/2 -> Terminator1/1

== system Last_Model_Interior_team/Switching/30_deg_Dpwm/Sector5/Enabled Subsystem ==
  Vabc : Inport
  Enable : EnablePort
  Add : Sum  Inputs=-+
  Constant : Constant  Value=-1
  Demux : Demux  Outputs=3
  Terminator : Terminator
  Terminator1 : Terminator
  Out1 : Outport
  wires:
  Demux/3 -> Terminator1/1
  Add/1 -> Out1/1
  Demux/1 -> Add/1
  Vabc/1 -> Demux/1
  Constant/1 -> Add/2
  Demux/2 -> Terminator/1

== system Last_Model_Interior_team/Switching/30_deg_Dpwm/Sector5/Enabled Subsystem1 ==
  Vabc : Inport
  Enable : EnablePort
  Add : Sum  Inputs=-+
  Constant : Constant
  Demux : Demux  Outputs=3
  Terminator : Terminator
  Terminator1 : Terminator
  Out1 : Outport
  wires:
  Demux/3 -> Add/1
  Add/1 -> Out1/1
  Constant/1 -> Add/2
  Demux/2 -> Terminator/1
  Vabc/1 -> Demux/1
  Demux/1 -> Terminator1/1

== system Last_Model_Interior_team/Switching/30_deg_Dpwm/Sector6/Enabled Subsystem ==
  Vabc : Inport
  Enable : EnablePort
  Add : Sum  Inputs=-+
  Constant : Constant  Value=-1
  Demux : Demux  Outputs=3
  Terminator : Terminator
  Terminator1 : Terminator
  Out1 : Outport
  wires:
  Demux/2 -> Terminator/1
  Constant/1 -> Add/2
  Vabc/1 -> Demux/1
  Demux/1 -> Add/1
  Add/1 -> Out1/1
  Demux/3 -> Terminator1/1

== system Last_Model_Interior_team/Switching/30_deg_Dpwm/Sector6/Enabled Subsystem1 ==
  Vabc : Inport
  Enable : EnablePort
  Add : Sum  Inputs=-+
  Constant : Constant
  Demux : Demux  Outputs=3
  Terminator : Terminator
  Terminator1 : Terminator
  Out1 : Outport
  wires:
  Vabc/1 -> Demux/1
  Demux/2 -> Add/1
  Constant/1 -> Add/2
  Add/1 -> Out1/1
  Demux/3 -> Terminator1/1
  Demux/1 -> Terminator/1

== system Last_Model_Interior_team/Switching/60deg_+30_shifted/Sector1/Enabled Subsystem ==
  Vabc : Inport
  Enable : EnablePort
  Add : Sum  Inputs=-+
  Constant : Constant
  Demux : Demux  Outputs=3
  Terminator : Terminator
  Terminator1 : Terminator
  Out1 : Outport
  wires:
  Demux/1 -> Terminator/1
  Constant/1 -> Add/2
  Vabc/1 -> Demux/1
  Demux/3 -> Terminator1/1
  Demux/2 -> Add/1
  Add/1 -> Out1/1

== system Last_Model_Interior_team/Switching/60deg_+30_shifted/Sector1/Enabled Subsystem1 ==
  Vabc : Inport
  Enable : EnablePort
  Add : Sum  Inputs=-+
  Constant : Constant
  Demux : Demux  Outputs=3
  Terminator : Terminator
  Terminator1 : Terminator
  Out1 : Outport
  wires:
  Add/1 -> Out1/1
  Demux/3 -> Terminator1/1
  Vabc/1 -> Demux/1
  Demux/2 -> Add/1
  Constant/1 -> Add/2
  Demux/1 -> Terminator/1

== system Last_Model_Interior_team/Switching/60deg_+30_shifted/Sector2/Enabled Subsystem ==
  Vabc : Inport
  Enable : EnablePort
  Add : Sum  Inputs=-+
  Constant : Constant  Value=-1
  Demux : Demux  Outputs=3
  Terminator : Terminator
  Terminator1 : Terminator
  Out1 : Outport
  wires:
  Add/1 -> Out1/1
  Vabc/1 -> Demux/1
  Demux/3 -> Add/1
  Constant/1 -> Add/2
  Demux/2 -> Terminator1/1
  Demux/1 -> Terminator/1

== system Last_Model_Interior_team/Switching/60deg_+30_shifted/Sector2/Enabled Subsystem1 ==
  Vabc : Inport
  Enable : EnablePort
  Add : Sum  Inputs=-+
  Constant : Constant  Value=-1
  Demux : Demux  Outputs=3
  Terminator : Terminator
  Terminator1 : Terminator
  Out1 : Outport
  wires:
  Demux/3 -> Add/1
  Vabc/1 -> Demux/1
  Demux/2 -> Terminator1/1
  Constant/1 -> Add/2
  Demux/1 -> Terminator/1
  Add/1 -> Out1/1

== system Last_Model_Interior_team/Switching/60deg_+30_shifted/Sector3/Enabled Subsystem ==
  Vabc : Inport
  Enable : EnablePort
  Add : Sum  Inputs=-+
  Constant : Constant
  Demux : Demux  Outputs=3
  Terminator : Terminator
  Terminator1 : Terminator
  Out1 : Outport
  wires:
  Demux/1 -> Add/1
  Demux/2 -> Terminator/1
  Constant/1 -> Add/2
  Vabc/1 -> Demux/1
  Demux/3 -> Terminator1/1
  Add/1 -> Out1/1

== system Last_Model_Interior_team/Switching/60deg_+30_shifted/Sector3/Enabled Subsystem1 ==
  Vabc : Inport
  Enable : EnablePort
  Add : Sum  Inputs=-+
  Constant : Constant
  Demux : Demux  Outputs=3
  Terminator : Terminator
  Terminator1 : Terminator
  Out1 : Outport
  wires:
  Add/1 -> Out1/1
  Demux/3 -> Terminator1/1
  Vabc/1 -> Demux/1
  Constant/1 -> Add/2
  Demux/2 -> Terminator/1
  Demux/1 -> Add/1

== system Last_Model_Interior_team/Switching/60deg_+30_shifted/Sector4/Enabled Subsystem ==
  Vabc : Inport
  Enable : EnablePort
  Add : Sum  Inputs=-+
  Constant : Constant  Value=-1
  Demux : Demux  Outputs=3
  Terminator : Terminator
  Terminator1 : Terminator
  Out1 : Outport
  wires:
  Add/1 -> Out1/1
  Vabc/1 -> Demux/1
  Demux/1 -> Terminator/1
  Constant/1 -> Add/2
  Demux/3 -> Terminator1/1
  Demux/2 -> Add/1

== system Last_Model_Interior_team/Switching/60deg_+30_shifted/Sector4/Enabled Subsystem1 ==
  Vabc : Inport
  Enable : EnablePort
  Add : Sum  Inputs=-+
  Constant : Constant  Value=-1
  Demux : Demux  Outputs=3
  Terminator : Terminator
  Terminator1 : Terminator
  Out1 : Outport
  wires:
  Demux/2 -> Add/1
  Demux/3 -> Terminator1/1
  Add/1 -> Out1/1
  Constant/1 -> Add/2
  Demux/1 -> Terminator/1
  Vabc/1 -> Demux/1

== system Last_Model_Interior_team/Switching/60deg_+30_shifted/Sector5/Enabled Subsystem ==
  Vabc : Inport
  Enable : EnablePort
  Add : Sum  Inputs=-+
  Constant : Constant
  Demux : Demux  Outputs=3
  Terminator : Terminator
  Terminator1 : Terminator
  Out1 : Outport
  wires:
  Demux/1 -> Terminator1/1
  Demux/2 -> Terminator/1
  Constant/1 -> Add/2
  Vabc/1 -> Demux/1
  Demux/3 -> Add/1
  Add/1 -> Out1/1

== system Last_Model_Interior_team/Switching/60deg_+30_shifted/Sector5/Enabled Subsystem1 ==
  Vabc : Inport
  Enable : EnablePort
  Add : Sum  Inputs=-+
  Constant : Constant
  Demux : Demux  Outputs=3
  Terminator : Terminator
  Terminator1 : Terminator
  Out1 : Outport
  wires:
  Demux/3 -> Add/1
  Vabc/1 -> Demux/1
  Demux/2 -> Terminator/1
  Demux/1 -> Terminator1/1
  Constant/1 -> Add/2
  Add/1 -> Out1/1

== system Last_Model_Interior_team/Switching/60deg_+30_shifted/Sector6/Enabled Subsystem ==
  Vabc : Inport
  Enable : EnablePort
  Add : Sum  Inputs=-+
  Constant : Constant  Value=-1
  Demux : Demux  Outputs=3
  Terminator : Terminator
  Terminator1 : Terminator
  Out1 : Outport
  wires:
  Add/1 -> Out1/1
  Demux/1 -> Add/1
  Demux/3 -> Terminator1/1
  Constant/1 -> Add/2
  Vabc/1 -> Demux/1
  Demux/2 -> Terminator/1

== system Last_Model_Interior_team/Switching/60deg_+30_shifted/Sector6/Enabled Subsystem1 ==
  Vabc : Inport
  Enable : EnablePort
  Add : Sum  Inputs=-+
  Constant : Constant  Value=-1
  Demux : Demux  Outputs=3
  Terminator : Terminator
  Terminator1 : Terminator
  Out1 : Outport
  wires:
  Demux/2 -> Terminator/1
  Demux/3 -> Terminator1/1
  Add/1 -> Out1/1
  Constant/1 -> Add/2
  Demux/1 -> Add/1
  Vabc/1 -> Demux/1

== system Last_Model_Interior_team/Switching/60deg_-30_shifted/Sector1/Enabled Subsystem ==
  Vabc : Inport
  Enable : EnablePort
  Add : Sum  Inputs=-+
  Constant : Constant
  Demux : Demux  Outputs=3
  Terminator : Terminator
  Terminator1 : Terminator
  Out1 : Outport
  wires:
  Add/1 -> Out1/1
  Demux/2 -> Add/1
  Demux/3 -> Terminator1/1
  Vabc/1 -> Demux/1
  Constant/1 -> Add/2
  Demux/1 -> Terminator/1

== system Last_Model_Interior_team/Switching/60deg_-30_shifted/Sector1/Enabled Subsystem1 ==
  Vabc : Inport
  Enable : EnablePort
  Add : Sum  Inputs=-+
  Constant : Constant
  Demux : Demux  Outputs=3
  Terminator : Terminator
  Terminator1 : Terminator
  Out1 : Outport
  wires:
  Demux/1 -> Terminator/1
  Constant/1 -> Add/2
  Demux/2 -> Add/1
  Vabc/1 -> Demux/1
  Demux/3 -> Terminator1/1
  Add/1 -> Out1/1

== system Last_Model_Interior_team/Switching/60deg_-30_shifted/Sector2/Enabled Subsystem ==
  Vabc : Inport
  Enable : EnablePort
  Add : Sum  Inputs=-+
  Constant : Constant  Value=-1
  Demux : Demux  Outputs=3
  Terminator : Terminator
  Terminator1 : Terminator
  Out1 : Outport
  wires:
  Demux/1 -> Terminator/1
  Demux/2 -> Terminator1/1
  Constant/1 -> Add/2
  Demux/3 -> Add/1
  Vabc/1 -> Demux/1
  Add/1 -> Out1/1

== system Last_Model_Interior_team/Switching/60deg_-30_shifted/Sector2/Enabled Subsystem1 ==
  Vabc : Inport
  Enable : EnablePort
  Add : Sum  Inputs=-+
  Constant : Constant  Value=-1
  Demux : Demux  Outputs=3
  Terminator : Terminator
  Terminator1 : Terminator
  Out1 : Outport
  wires:
  Add/1 -> Out1/1
  Demux/1 -> Terminator/1
  Constant/1 -> Add/2
  Demux/2 -> Terminator1/1
  Vabc/1 -> Demux/1
  Demux/3 -> Add/1

== system Last_Model_Interior_team/Switching/60deg_-30_shifted/Sector3/Enabled Subsystem ==
  Vabc : Inport
  Enable : EnablePort
  Add : Sum  Inputs=-+
  Constant : Constant
  Demux : Demux  Outputs=3
  Terminator : Terminator
  Terminator1 : Terminator
  Out1 : Outport
  wires:
  Add/1 -> Out1/1
  Demux/3 -> Terminator1/1
  Vabc/1 -> Demux/1
  Constant/1 -> Add/2
  Demux/2 -> Terminator/1
  Demux/1 -> Add/1

== system Last_Model_Interior_team/Switching/60deg_-30_shifted/Sector3/Enabled Subsystem1 ==
  Vabc : Inport
  Enable : EnablePort
  Add : Sum  Inputs=-+
  Constant : Constant
  Demux : Demux  Outputs=3
  Terminator : Terminator
  Terminator1 : Terminator
  Out1 : Outport
  wires:
  Demux/1 -> Add/1
  Demux/2 -> Terminator/1
  Constant/1 -> Add/2
  Vabc/1 -> Demux/1
  Demux/3 -> Terminator1/1
  Add/1 -> Out1/1

== system Last_Model_Interior_team/Switching/60deg_-30_shifted/Sector4/Enabled Subsystem ==
  Vabc : Inport
  Enable : EnablePort
  Add : Sum  Inputs=-+
  Constant : Constant  Value=-1
  Demux : Demux  Outputs=3
  Terminator : Terminator
  Terminator1 : Terminator
  Out1 : Outport
  wires:
  Demux/2 -> Add/1
  Demux/3 -> Terminator1/1
  Constant/1 -> Add/2
  Demux/1 -> Terminator/1
  Vabc/1 -> Demux/1
  Add/1 -> Out1/1

== system Last_Model_Interior_team/Switching/60deg_-30_shifted/Sector4/Enabled Subsystem1 ==
  Vabc : Inport
  Enable : EnablePort
  Add : Sum  Inputs=-+
  Constant : Constant  Value=-1
  Demux : Demux  Outputs=3
  Terminator : Terminator
  Terminator1 : Terminator
  Out1 : Outport
  wires:
  Vabc/1 -> Demux/1
  Demux/1 -> Terminator/1
  Constant/1 -> Add/2
  Add/1 -> Out1/1
  Demux/3 -> Terminator1/1
  Demux/2 -> Add/1

== system Last_Model_Interior_team/Switching/60deg_-30_shifted/Sector5/Enabled Subsystem ==
  Vabc : Inport
  Enable : EnablePort
  Add : Sum  Inputs=-+
  Constant : Constant
  Demux : Demux  Outputs=3
  Terminator : Terminator
  Terminator1 : Terminator
  Out1 : Outport
  wires:
  Add/1 -> Out1/1
  Demux/3 -> Add/1
  Vabc/1 -> Demux/1
  Constant/1 -> Add/2
  Demux/2 -> Terminator/1
  Demux/1 -> Terminator1/1

== system Last_Model_Interior_team/Switching/60deg_-30_shifted/Sector5/Enabled Subsystem1 ==
  Vabc : Inport
  Enable : EnablePort
  Add : Sum  Inputs=-+
  Constant : Constant
  Demux : Demux  Outputs=3
  Terminator : Terminator
  Terminator1 : Terminator
  Out1 : Outport
  wires:
  Add/1 -> Out1/1
  Constant/1 -> Add/2
  Demux/1 -> Terminator1/1
  Demux/2 -> Terminator/1
  Vabc/1 -> Demux/1
  Demux/3 -> Add/1

== system Last_Model_Interior_team/Switching/60deg_-30_shifted/Sector6/Enabled Subsystem ==
  Vabc : Inport
  Enable : EnablePort
  Add : Sum  Inputs=-+
  Constant : Constant  Value=-1
  Demux : Demux  Outputs=3
  Terminator : Terminator
  Terminator1 : Terminator
  Out1 : Outport
  wires:
  Demux/2 -> Terminator/1
  Vabc/1 -> Demux/1
  Constant/1 -> Add/2
  Demux/3 -> Terminator1/1
  Demux/1 -> Add/1
  Add/1 -> Out1/1

== system Last_Model_Interior_team/Switching/60deg_-30_shifted/Sector6/Enabled Subsystem1 ==
  Vabc : Inport
  Enable : EnablePort
  Add : Sum  Inputs=-+
  Constant : Constant  Value=-1
  Demux : Demux  Outputs=3
  Terminator : Terminator
  Terminator1 : Terminator
  Out1 : Outport
  wires:
  Vabc/1 -> Demux/1
  Demux/1 -> Add/1
  Constant/1 -> Add/2
  Add/1 -> Out1/1
  Demux/3 -> Terminator1/1
  Demux/2 -> Terminator/1

== system Last_Model_Interior_team/Switching/60deg_DPWM/Sector1/Enabled Subsystem ==
  Vabc : Inport
  Enable : EnablePort
  Add : Sum  Inputs=-+
  Constant : Constant
  Demux : Demux  Outputs=3
  Terminator : Terminator
  Terminator1 : Terminator
  Out1 : Outport
  wires:
  Demux/1 -> Terminator/1
  Constant/1 -> Add/2
  Vabc/1 -> Demux/1
  Demux/3 -> Terminator1/1
  Demux/2 -> Add/1
  Add/1 -> Out1/1
